simulink model "sistema_termicosim"  (R2023a)
settings: Solver=VariableStepAuto  StartTime=0.0  StopTime=30  RelTol=1e-3
model workspace (MAT data in the model file):
  algo = 1
settings Model: Creator=Fabian  LastModifiedBy=ML026
settings SolverCC: AlgebraicLoopSolver=TrustRegion
settings DebuggingCC: UnconnectedInputMsg=warning  UnconnectedOutputMsg=warning  UnconnectedLineMsg=warning
settings ModelReferenceCC: EnableRefExpFcnMdlSchedulingChecks=on

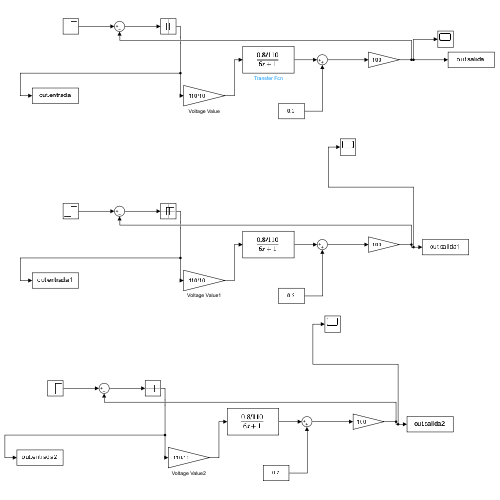
[thumbnail: Simulink's stored preview of the top-level diagram]
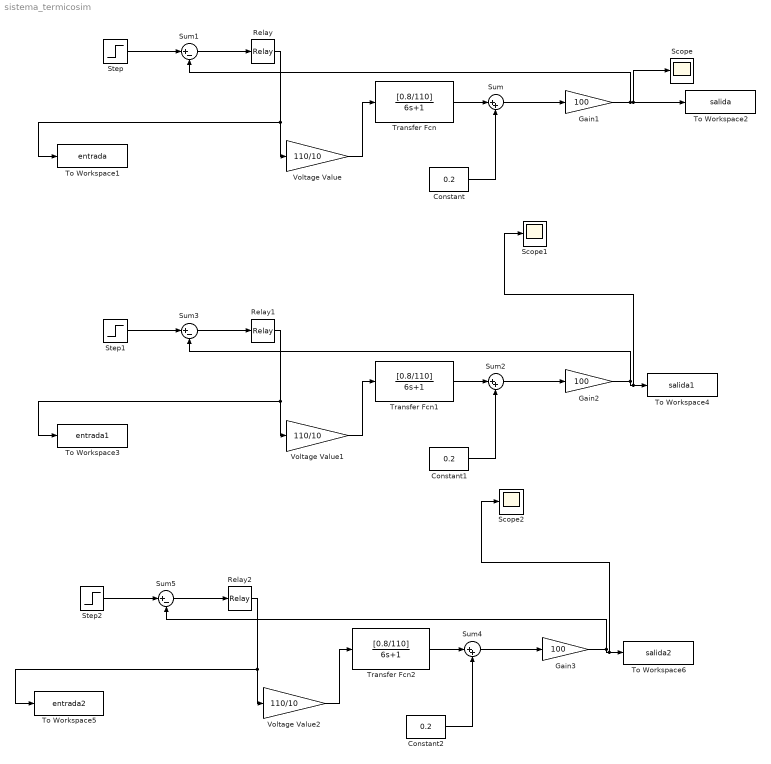
== system sistema_termicosim ==
  Constant : Constant  Value=0.2  VectorParams1D=off
  Constant1 : Constant  Value=0.2  VectorParams1D=off
  Constant2 : Constant  Value=0.2  VectorParams1D=off
  Gain1 : Gain  Gain=100
  Gain2 : Gain  Gain=100
  Gain3 : Gain  Gain=100
  Relay : Relay  OnSwitchValue=20  OffSwitchValue=-20  OnOutputValue=10
  Relay1 : Relay  OnSwitchValue=5  OffSwitchValue=-5  OnOutputValue=10
  Relay2 : Relay  OnSwitchValue=1  OffSwitchValue=-1  OnOutputValue=10
  Scope : Scope
  Scope1 : Scope
  Scope2 : Scope
  Step : Step  Time=0  After=50  SampleTime=0
  Step1 : Step  Time=0  After=45  SampleTime=0
  Step2 : Step  Time=0  After=40  SampleTime=0
  Sum : Sum  Inputs=|++
  Sum1 : Sum  Inputs=|+-
  Sum2 : Sum  Inputs=|++
  Sum3 : Sum  Inputs=|+-
  Sum4 : Sum  Inputs=|++
  Sum5 : Sum  Inputs=|+-
  To Workspace1 : ToWorkspace  VariableName=entrada  SaveFormat=Timeseries  SampleTime=-1
  To Workspace2 : ToWorkspace  VariableName=salida  SaveFormat=Timeseries  SampleTime=-1
  To Workspace3 : ToWorkspace  VariableName=entrada1  SaveFormat=Timeseries  SampleTime=-1
  To Workspace4 : ToWorkspace  VariableName=salida1  SaveFormat=Timeseries  SampleTime=-1
  To Workspace5 : ToWorkspace  VariableName=entrada2  SaveFormat=Timeseries  SampleTime=-1
  To Workspace6 : ToWorkspace  VariableName=salida2  SaveFormat=Timeseries  SampleTime=-1
  Transfer Fcn : TransferFcn  Numerator=[0.8/110]  Denominator=[6 1]
  Transfer Fcn1 : TransferFcn  Numerator=[0.8/110]  Denominator=[6 1]
  Transfer Fcn2 : TransferFcn  Numerator=[0.8/110]  Denominator=[6 1]
  Voltage Value : Gain  Gain=110/10
  Voltage Value1 : Gain  Gain=110/10
  Voltage Value2 : Gain  Gain=110/10
  wires:
  Transfer Fcn/1 -> Sum/1
  Constant/1 -> Sum/2
  Voltage Value/1 -> Transfer Fcn/1
  Gain1/1 -> Scope/1, To Workspace2/1, Sum1/2
  Sum/1 -> Gain1/1
  Step/1 -> Sum1/1
  Sum1/1 -> Relay/1
  Relay/1 -> To Workspace1/1, Voltage Value/1
  Sum2/1 -> Gain2/1
  Voltage Value1/1 -> Transfer Fcn1/1
  Transfer Fcn1/1 -> Sum2/1
  Gain2/1 -> Scope1/1, To Workspace4/1, Sum3/2
  Step1/1 -> Sum3/1
  Constant1/1 -> Sum2/2
  Sum3/1 -> Relay1/1
  Relay1/1 -> To Workspace3/1, Voltage Value1/1
  Relay2/1 -> To Workspace5/1, Voltage Value2/1
  Sum5/1 -> Relay2/1
  Constant2/1 -> Sum4/2
  Sum4/1 -> Gain3/1
  Step2/1 -> Sum5/1
  Transfer Fcn2/1 -> Sum4/1
  Voltage Value2/1 -> Transfer Fcn2/1
  Gain3/1 -> Scope2/1, To Workspace6/1, Sum5/2
